simulink model "tcp_client"  (R2022b)
settings: Solver=ode3  StartTime=0.0  StopTime=15  FixedStep=0.1  RelTol=1e-3
settings Model: Creator=yaozhong.zhang  LastModifiedBy=91703
settings SolverCC: AlgebraicLoopSolver=TrustRegion
settings DebuggingCC: UnconnectedInputMsg=warning  UnconnectedOutputMsg=warning  UnconnectedLineMsg=warning  SFMachineParentedDataDiag=warning
settings ModelReferenceCC: EnableRefExpFcnMdlSchedulingChecks=on

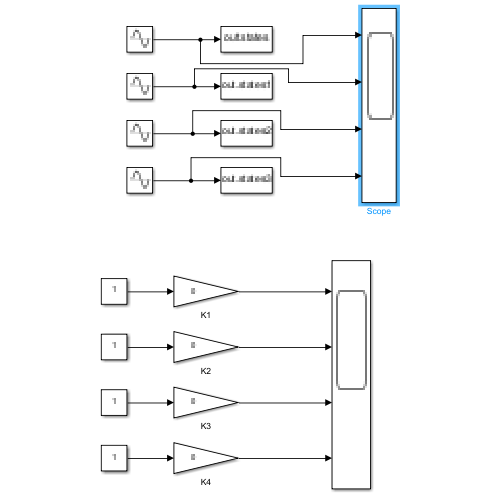
[thumbnail: Simulink's stored preview of the top-level diagram]
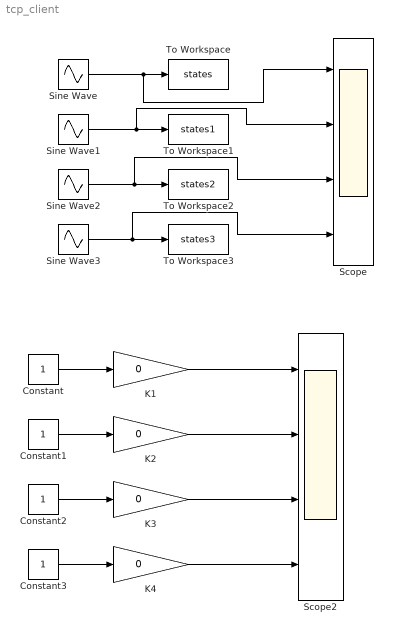
== system tcp_client ==
  Constant{,1..3} (4 alike) : Constant
  K{1..4} (4 alike) : Gain  Gain=0
  Scope : Scope  NumInputPorts=4
  Scope2 : Scope  NumInputPorts=4
  Sine Wave : Sin  SampleTime=0
  Sine Wave1 : Sin  Phase=pi/2  SampleTime=0
  Sine Wave2 : Sin  Phase=pi  SampleTime=0
  Sine Wave3 : Sin  Phase=3*pi/2  SampleTime=0
  To Workspace : ToWorkspace  VariableName=states  SaveFormat=Timeseries  SampleTime=-1
  To Workspace1 : ToWorkspace  VariableName=states1  SaveFormat=Timeseries  SampleTime=-1
  To Workspace2 : ToWorkspace  VariableName=states2  SaveFormat=Timeseries  SampleTime=-1
  To Workspace3 : ToWorkspace  VariableName=states3  SaveFormat=Timeseries  SampleTime=-1
  wires:
  Constant1/1 -> K2/1
  K3/1 -> Scope2/3
  Constant/1 -> K1/1
  Constant2/1 -> K3/1
  K2/1 -> Scope2/2
  K1/1 -> Scope2/1
  Sine Wave/1 -> Scope/1, To Workspace/1
  Sine Wave1/1 -> Scope/2, To Workspace1/1
  Sine Wave2/1 -> Scope/3, To Workspace2/1
  Sine Wave3/1 -> Scope/4, To Workspace3/1
  Constant3/1 -> K4/1
  K4/1 -> Scope2/4
